simulink model "bbt_pid_hg_sl"  (Simulink 7.9)
settings: Solver=FixedStepDiscrete  SolverMode=SingleTasking  StartTime=0.0  StopTime=inf  RelTol=1e-3
values from neighbouring files (symbols this model uses):
  K_theta_hg = (pi/180)*(2.1/15)    (= 0.00244346095279)    [bbt_lqr_hg.m]    (also in bbt_lqr_servo_hg.m; bbt_pid_hg.m)
  Kd = (-(p1+p2)*T - 1)/K    [bbt_pid_hg.m]    (also in sim_param.mat = 0)
  kd = -(p1+p2+p3)/K_b    [bbt_pid_hg.m]
  kff = ki/alpha    [bbt_pid_hg.m]
  ki = -p1*p2*p3/K_b    [bbt_pid_hg.m]
  Kp = p1*p2*T/K    [bbt_pid_hg.m]    (also in sim_param.mat = 0)
  kp = (p1*p2 + p2*p3 + p3*p1)/K_b    [bbt_pid_hg.m]
  r = 60    [sim_param.mat]
  r1 = 20    [bbt_lqr_hg.m]    (also in bbt_lqr_servo_hg.m = 15; bbt_pid_hg.m = 15)
  r2 = 20    [bbt_lqr_hg.m]    (also in bbt_lqr_servo_hg.m = 25; bbt_pid_hg.m = 25)
  r_cyc = 4    [sim_param.mat]
  ts = 0.02    [sim_param.mat]
undefined symbols (not defined in the file or in its folder): denlpf, DiscIntNeverNeededParam, numlpf
libraries: simulink x5, arduinolib x4
settings Model: Creator=hirata  LastModifiedBy=hirata  SimulationMode=external  ExtModeTrigDuration=2
settings OptimizationCC: OptimizeModelRefInitCode=on  LifeSpan=1
settings DebuggingCC: SolverPrmCheckMsg=none  StrictBusMsg=Warning
settings HardwareCC: ProdBitPerInt=16  ProdBitPerPointer=8  ProdIntDivRoundTo=Zero  ProdEndianess=LittleEndian  ProdWordSize=8  ProdHWDeviceType=Atmel->AVR
settings RTWCC: SystemTargetFile=realtime.tlc  GenerateMakefile=off  TemplateMakefile=realtime.tmf  Description=Real-Time Toolbox  RTWVerbose=off  ProcessScript=realtime_make_rtw_hook
settings STFCustomTargetCC: TargetLibSuffix=.a  CodeReplacementLibrary=ANSI_C  GenerateSampleERTMain=on  ERTCustomFileBanners=on  SupportNonInlinedSFcns=off  SupportVariableSizeSignals=on  GRTInterface=off  SystemTargetFile=realtime.tlc
settings ERTTargetCC: CodeReplacementLibrary=ANSI_C  MultiwordLength=2048  GenerateSampleERTMain=on  ParMdlRefBuildCompliant=off  CompOptLevelCompliant=off  ConcurrentExecutionCompliant=off  CombineOutputUpdateFcns=off  ERTFirstTimeCompliant=off  SupportContinuousTime=on  SupportVariableSizeSignals=on  ModelStepFunctionPrototypeControlCompliant=off  CPPClassGenCompliant=off  ExtMode=on  ExtModeTransport=3  ExtModeMexFile=ext_serial_win32_comm  ExtModeMexArgs=0 3 115200  InlinedParameterPlacement=NonHierarchical  ERTSrcFileBannerTemplate=realtime_code_template.cgt  ERTHdrFileBannerTemplate=realtime_code_template.cgt  ERTDataSrcFileTemplate=realtime_code_template.cgt  ERTDataHdrFileTemplate=realtime_code_template.cgt  ERTCustomFileTemplate=realtime_file_process.tlc  ConvertIfToSwitch=off  SuppressUnreachableDefaultCases=off
settings SettingsController: Description=Run on Hardware Dialog  TargetExtensionPlatform=Arduino Mega 2560
settings MATStruct: Set_host_COM_port=[0.0]  COM_port_number=1  COM_port_baud_rate=115200  Enable_overrun_detection=[0.0]  Digital_output_to_set_on_overrun=13  Analog_input_reference_voltage=[0.0]  Serial0_baud_rate=9600  Serial1_baud_rate=9600  Serial2_baud_rate=9600  Serial3_baud_rate=9600

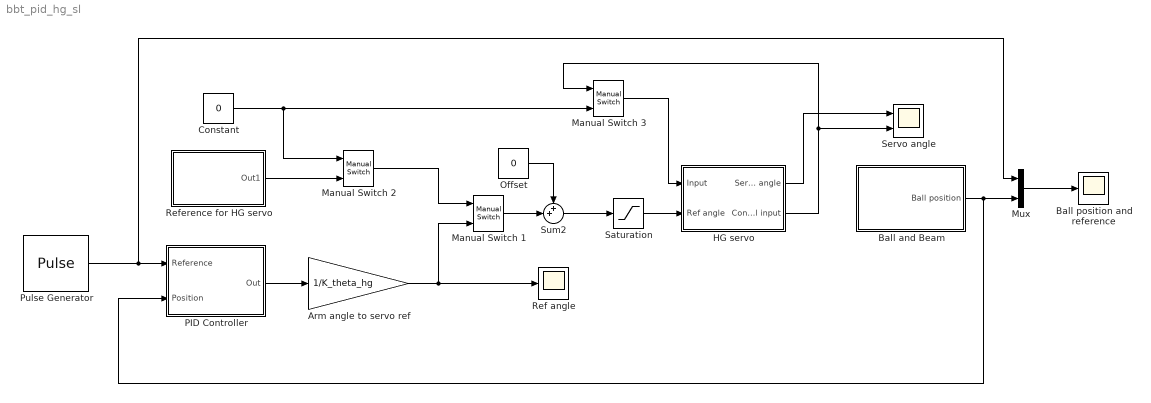
== system bbt_pid_hg_sl ==
  Arm angle to servo ref : Gain  Gain=1/K_theta_hg
  Ball and Beam : Subsystem
  Ball position and reference : Scope
      settings: TimeRange=30  YMin=-15  YMax=25
  Constant : Constant  Value=0
  HG servo : Subsystem
  Manual Switch 1 : simulink/Signal Routing/Manual Switch  sw=0  action=0  varsize=off
  Manual Switch 2 : simulink/Signal Routing/Manual Switch  sw=1  action=0  varsize=off
  Manual Switch 3 : simulink/Signal Routing/Manual Switch  sw=0  action=0  varsize=off
  Mux : Mux  Inputs=2
  Offset : Constant  Value=0  SampleTime=ts
  PID Controller : Subsystem
  Pulse Generator : DiscretePulseGenerator  PulseType=Time based  Amplitude=r2-r1  Period=30  PulseWidth=50  PhaseDelay=10
  Ref angle : Scope
      settings: TimeRange=30  YMin=-40  YMax=40  SaveName=ScopeData5
  Reference for HG servo : Subsystem
  Saturation : Saturate  UpperLimit=45  LowerLimit=-45
  Servo angle : Scope  NumInputPorts=2
      settings: TimeRange=10  YMin=-50~-5  YMax=50~5  SaveName=ScopeData4
  Sum2 : Sum  Inputs=++|
  wires:
  Offset/1 -> Sum2/1
  Arm angle to servo ref/1 -> Manual Switch 1/2, Ref angle/1
  Sum2/1 -> Saturation/1
  Mux/1 -> Ball position and reference/1
  Manual Switch 1/1 -> Sum2/2
  Saturation/1 -> HG servo/2(Ref angle)
  Ball and Beam/1(Ball position) -> Mux/2, PID Controller/2(Position)
  Pulse Generator/1 -> Mux/1, PID Controller/1(Reference)
  PID Controller/1(Out) -> Arm angle to servo ref/1
  HG servo/1(Servo angle) -> Servo angle/1
  HG servo/2(Control input) -> Servo angle/2, Manual Switch 3/1
  Manual Switch 2/1 -> Manual Switch 1/1
  Reference for HG servo/1(Out1) -> Manual Switch 2/2
  Constant/1 -> Manual Switch 2/1, Manual Switch 3/2
  Manual Switch 3/1 -> HG servo/1(Input)

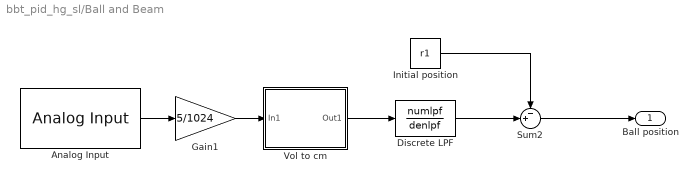
== system bbt_pid_hg_sl/Ball and Beam ==
  Analog Input : arduinolib/Analog Input  pinNumber=2  sampleTime=ts
  Discrete LPF : DiscreteTransferFcn  Numerator=numlpf  Denominator=denlpf
  Gain1 : Gain  Gain=5/1024
  Initial position : Constant  Value=r1
  Sum2 : Sum  Inputs=-+|
  Vol to cm : Subsystem
  Ball position : Outport
  wires:
  Analog Input/1 -> Gain1/1
  Gain1/1 -> Vol to cm/1(In1)
  Vol to cm/1(Out1) -> Discrete LPF/1
  Initial position/1 -> Sum2/1
  Discrete LPF/1 -> Sum2/2
  Sum2/1 -> Ball position/1

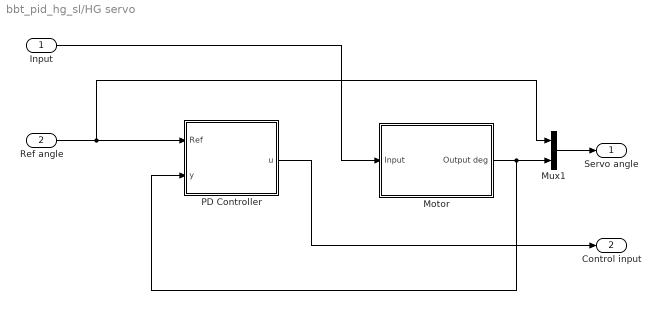
== system bbt_pid_hg_sl/HG servo ==
  Input : Inport
  Ref angle : Inport  Port=2
  Motor : Subsystem
  Mux1 : Mux  Inputs=2
  PD Controller : Subsystem
  Servo angle : Outport
  Control input : Outport  Port=2
  wires:
  Mux1/1 -> Servo angle/1
  Motor/1(Output deg) -> Mux1/2, PD Controller/2(y)
  Ref angle/1 -> Mux1/1, PD Controller/1(Ref)
  PD Controller/1(u) -> Control input/1
  Input/1 -> Motor/1(Input)

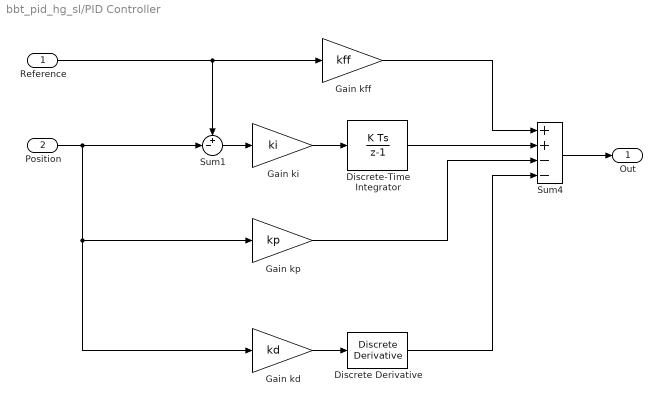
== system bbt_pid_hg_sl/PID Controller ==
  Reference : Inport
  Position : Inport  Port=2
  Discrete Derivative : simulink/Discrete/Discrete Derivative  gainval=1.0  ICPrevScaledInput=0.0  InputProcessing=Inherited  OutMin=[]  OutMax=[]  OutDataType=fixdt(1, 16)  OutScaling=2^-10  DoSatur=off
  Discrete-Time Integrator : DiscreteIntegrator  SampleTime=ts  LimitOutput=on  UpperSaturationLimit=0.05  LowerSaturationLimit=-0.05  ICPrevOutput=DiscIntNeverNeededParam  ICPrevScaledInput=DiscIntNeverNeededParam
  Gain kd : Gain  Gain=kd
  Gain kff : Gain  Gain=kff
  Gain ki : Gain  Gain=ki
  Gain kp : Gain  Gain=kp
  Sum1 : Sum  Inputs=+-|
  Sum4 : Sum  Inputs=++--
  Out : Outport
  wires:
  Reference/1 -> Sum1/1, Gain kff/1
  Sum1/1 -> Gain ki/1
  Position/1 -> Sum1/2, Gain kp/1, Gain kd/1
  Discrete-Time Integrator/1 -> Sum4/2
  Gain ki/1 -> Discrete-Time Integrator/1
  Sum4/1 -> Out/1
  Gain kff/1 -> Sum4/1
  Gain kp/1 -> Sum4/3
  Gain kd/1 -> Discrete Derivative/1
  Discrete Derivative/1 -> Sum4/4

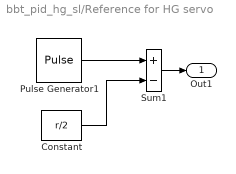
== system bbt_pid_hg_sl/Reference for HG servo ==
  Constant : Constant  Value=r/2
  Pulse Generator1 : DiscretePulseGenerator  PulseType=Time based  Amplitude=r  Period=r_cyc  PulseWidth=50
  Sum1 : Sum  Inputs=+-
  Out1 : Outport
  wires:
  Pulse Generator1/1 -> Sum1/1
  Constant/1 -> Sum1/2
  Sum1/1 -> Out1/1

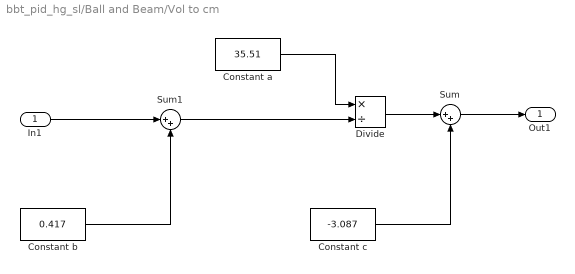
== system bbt_pid_hg_sl/Ball and Beam/Vol to cm ==
  In1 : Inport
  Constant a : Constant  Value=35.51
  Constant b : Constant  Value=0.417
  Constant c : Constant  Value=-3.087
  Divide : Product  Inputs=*/
  Sum : Sum  Inputs=|++
  Sum1 : Sum  Inputs=|++
  Out1 : Outport
  wires:
  Constant a/1 -> Divide/1
  Divide/1 -> Sum/1
  Sum/1 -> Out1/1
  Constant c/1 -> Sum/2
  In1/1 -> Sum1/1
  Sum1/1 -> Divide/2
  Constant b/1 -> Sum1/2

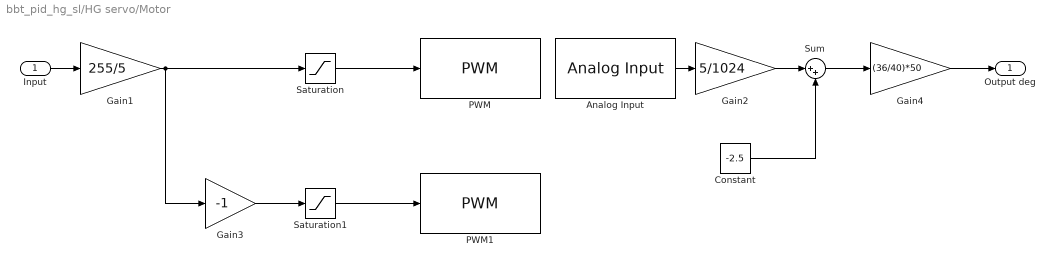
== system bbt_pid_hg_sl/HG servo/Motor ==
  Input : Inport
  Analog Input : arduinolib/Analog Input  pinNumber=0  sampleTime=ts
  Constant : Constant  Value=-2.5
  Gain1 : Gain  Gain=255/5
  Gain2 : Gain  Gain=5/1024
  Gain3 : Gain  Gain=-1
  Gain4 : Gain  Gain=(36/40)*50
  PWM : arduinolib/PWM  pinNumber=3
  PWM1 : arduinolib/PWM  pinNumber=5
  Saturation : Saturate  UpperLimit=255  LowerLimit=0
  Saturation1 : Saturate  UpperLimit=255  LowerLimit=0
  Sum : Sum  Inputs=|++
  Output deg : Outport
  wires:
  Gain3/1 -> Saturation1/1
  Constant/1 -> Sum/2
  Sum/1 -> Gain4/1
  Gain2/1 -> Sum/1
  Gain4/1 -> Output deg/1
  Saturation1/1 -> PWM1/1
  Gain1/1 -> Saturation/1, Gain3/1
  Saturation/1 -> PWM/1
  Analog Input/1 -> Gain2/1
  Input/1 -> Gain1/1

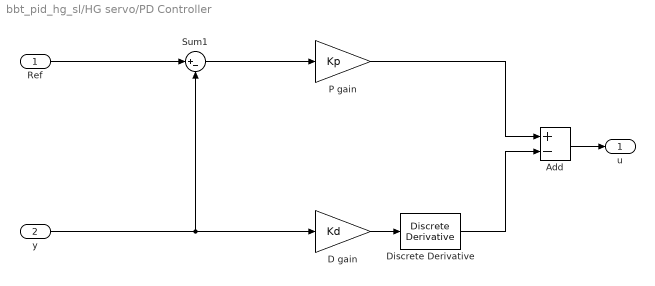
== system bbt_pid_hg_sl/HG servo/PD Controller ==
  Ref : Inport
  y : Inport  Port=2
  Add : Sum  Inputs=+-
  D gain : Gain  Gain=Kd
  Discrete Derivative : simulink/Discrete/Discrete Derivative  gainval=1.0  ICPrevScaledInput=0.0  InputProcessing=Inherited  OutMin=[]  OutMax=[]  OutDataType=fixdt(1, 16)  OutScaling=2^-10  DoSatur=off
  P gain : Gain  Gain=Kp
  Sum1 : Sum  Inputs=|+-
  u : Outport
  wires:
  D gain/1 -> Discrete Derivative/1
  Discrete Derivative/1 -> Add/2
  Add/1 -> u/1
  Ref/1 -> Sum1/1
  P gain/1 -> Add/1
  y/1 -> D gain/1, Sum1/2
  Sum1/1 -> P gain/1
